simulink model "AirRefueling_Platform_ch10_WindGust"  (R2022a)
settings: Solver=ode3  StartTime=0.0  StopTime=270  FixedStep=0.01  RelTol=1e-5  AbsTol=1e-4  EnableMultiTasking=on
InitFcn:
  | F16_Init
values from neighbouring files (symbols this model uses):
  airSpeed = 393.72    [F16_Init.m]
  alpha0 = trimAlpha*180/pi    (= 6.62393794015)    [F16_Init.m]
  altitude = 9843    [F16_Init.m]
  b_ref = 30.0    (= 30)    [F16_Init.m]
  C = [ 1,0,0,zeros(1,15) ... (first row only)    [F16_Init.m]
  C2m = [C(1,:) ... (first row only)    [F16_Init.m]
  d_f_rc = [4.45;0;-3.81]    [F16_Init.m]
  d_pr_rc = [8.2;0.45;-3.3]    [F16_Init.m]
  dLEF = 0    [F16_Init.m]
  fi_flag = 1    [F16_Init.m]
  Kc = [ ... (first row only)    [F16_Init.m]
  Ki = zeros(4,3)    [F16_Init.m]
  Kp = zeros(4,18)    [F16_Init.m]
  mass = 636.94    [F16_Init.m]
  p0_pr = p0_rc + d_pr_rc    [F16_Init.m]
  p0_rc = [-28;0;0]    [F16_Init.m]
  trim_ail = 0.00874607850103852    (= 0.00874607850104)    [F16_Init.m]
  trim_control = [trim_thrust;trim_ele;trim_ail;trim_rud]    [F16_Init.m]
  trim_ele = -2.97973164860638    (= -2.97973164861)    [F16_Init.m]
  trim_rud = 0.0680302158182712    (= 0.0680302158183)    [F16_Init.m]
  trim_state1 = [trim_state;0;0;0;0;0;0]    [F16_Init.m]
  trim_thrust = 2279.08519954656    (= 2279.08519955)    [F16_Init.m]
  visual_err = [0;0;0]    [F16_Init.m]
undefined symbols (not defined in the file or in its folder): Cdr_, dockingPoint, dtheta10, dtheta20, F, height, k_reel, kd, l0, l1, l_density, Light, m0, Mdr, MIL, N, Rdr, Rl, STD, T_reel_initial, theta10, theta20, vt0
libraries: etargetslib x11, dspnetwork x10, aerolibconvert2 x6, aerolibasang x4, simulink x2, aerolibatmos2 x2, aerolibwind2 x2, aerolibobsolete x2, sharedtransform x2, aerolibutil x2, aerolibadyn x1, aerolibtransform2 x1
(part 1 of 3)
settings Model: Creator=WhisPer  LastModifiedBy=lzj
settings SolverCC: AutoScaleAbsTol=off  AlgebraicLoopSolver=TrustRegion
settings DataIOCC: LimitDataPoints=on  SaveFormat=Array  ReturnWorkspaceOutputs=off
settings OptimizationCC: LifeSpan=inf
settings DebuggingCC: UnderspecifiedInitializationDetection=Classic  MergeDetectMultiDrivingBlocksExec=none  SolverPrmCheckMsg=warning  InheritedTsInSrcMsg=none  ParameterPrecisionLossMsg=none  UnconnectedInputMsg=warning  UnconnectedOutputMsg=warning  UnconnectedLineMsg=warning  StateNameClashWarn=warning  SFUnexpectedBacktrackingDiag=warning  SFNoUnconditionalDefaultTransitionDiag=warning  SFExecutionAtInitializationDiag=none  SFMachineParentedDataDiag=warning  ArithmeticOperatorsInVariantConditions=warning
settings HardwareCC: ProdBitPerPointer=32  ProdBitPerSizeT=32  ProdBitPerPtrDiffT=32  ProdLargestAtomicFloat=None  ProdIntDivRoundTo=Undefined  ProdEndianess=Unspecified  ProdWordSize=32  ProdHWDeviceType=32-bit Generic
settings ModelReferenceCC: PropagateSignalLabelsOutOfModel=off
settings SFSimCC: SimUseLocalCustomCode=off  CustomCodeUndefinedFunction=UseInterfaceOnly
settings RTWCC: RTWUseLocalCustomCode=off  DLArmComputeVersion=19.05
settings CodeAppCC: StateflowObjectComments=on
settings GRTTargetCC: TargetLangStandard=C89/C90 (ANSI)
settings ConfigComp: CovMetricSettings=dw  CovSaveCumulativeToWorkspaceVar=on  CovSaveSingleToWorkspaceVar=on  CovExternalEMLEnable=off

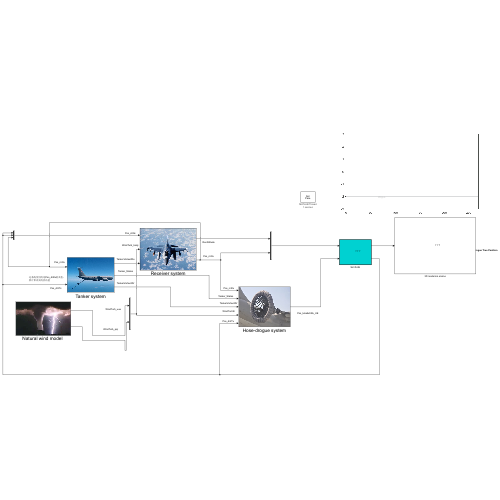
[thumbnail: Simulink's stored preview of the top-level diagram]
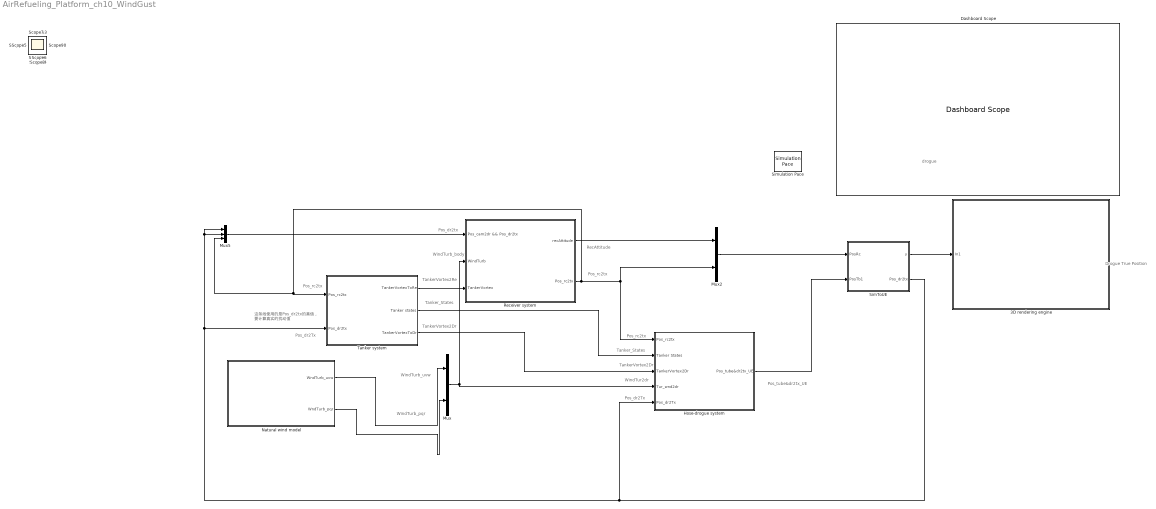
== system AirRefueling_Platform_ch10_WindGust ==
  note: 这条线使用的是Pos_dr2tx的真值，
      | 要计算真实的扰动值
  note: drogue
  note: RecAttitude
  note: WindTurb_uvw
  note: WindTurb_pqr
  note: Pos_tube&dr2tx_UE
  note: WindTur2dr
  note: WindTurb_body
  note: Pos_dr2tx
  note: Pos_rc2tx
  note: TankerVortex2Re
  note: TankerVortex2Dr
  note: Tanker_States
  note: Tanker_States
  note: TankerVortex2Dr
  note: Pos_rc2tx
  note: Drogue True Position
  note: Pos_dr2Tx
  note: Pos_rc2tx
  note: Pos_dr2Tx
  3D rendering engine : Subsystem
      mask Display: image('C:\Users\lgy13\Desktop\当下要完成的\AirRefueling3DVR-Blank\Icon\sideview.png'); % Use "Edit Image" on toolstrip to change.
  Dashboard Scope : DashboardScope
  Hose-drogue system : Subsystem
      mask Display: image(imread('Icon\drogue.jpg'))
  Mux : Mux  Inputs=2
  Mux2 : Mux  Inputs=2
  Mux5 : Mux  Inputs=3
  "Natural wind model " : Subsystem
      mask Display: image(imread('Icon\Enviroment.jpg'))
  Receiver system : Subsystem
      mask Display: image(imread('Icon\f16thumb.jpg'))
  SimToUE : MATLAB Function  TreatAsAtomicUnit=on
  Simulation Pace : aerolibanimutils/Simulation Pace  SimulationPace=1  SleepMode=MATLAB Thread  OutputPaceError=off  SampleTime=0.1
  Tanker system : Subsystem
      mask Display: image(imread('Icon\tanker.jpg'))
  Scope{,1,3..34} (34 alike) : Scope
  wires:
  SimToUE/2(Pos_dr2tx) -> Hose-drogue system/5(Pos_dr2Tx), Tanker system/2(Pos_dr2tx), Mux5/1, Mux5/2
  Receiver system/1(recAttitude) -> Mux2/1
  Hose-drogue system/1(Pos_tube&dr2tx_UE) -> SimToUE/2(PosTb1)
  Mux2/1 -> SimToUE/1(PosRc)
  Tanker system/2(Tanker states) -> Hose-drogue system/2(Tanker States)
  Tanker system/3(TankerVortexToDr) -> Hose-drogue system/3(TankerVortex2Dr)
  Tanker system/1(TankerVortexToRe) -> Receiver system/3(TankerVortex)
  Mux5/1 -> Receiver system/1(Pos_cam2dr && Pos_dr2tx)
  SimToUE/1(y) -> 3D rendering engine/1(In1)
  Receiver system/2(Pos_rc2tx) -> Mux2/2, Hose-drogue system/1(Pos_rc2tx), Mux5/3, Tanker system/1(Pos_rc2tx)
  "Natural wind model "/1(WndTurb_uvw) -> Mux/1
  "Natural wind model "/2(WndTurb_pqr) -> Mux/2
  Mux/1 -> Hose-drogue system/4(Tur_wnd2dr), Receiver system/2(WindTurb)

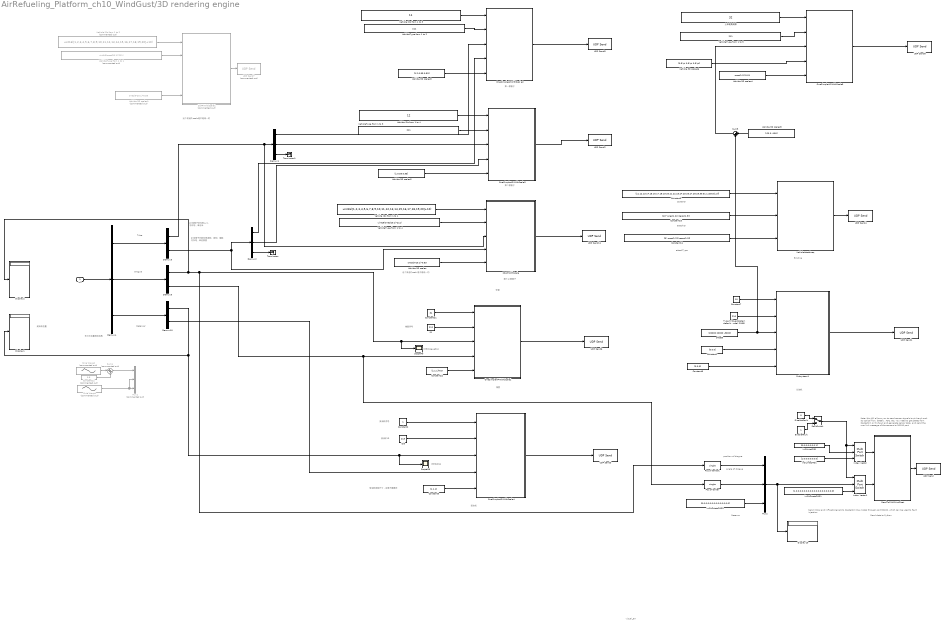
== system AirRefueling_Platform_ch10_WindGust/3D rendering engine ==
  note: visual_err
  note: 第一根管子
  note: 这个发送的scale是不是统一的
  note: 受油机位置
  note: 加油机
  note: 锥套
  note: position of drogue
  note: copterID
  note: Send inSILs and inFloats signals to CopterSim DLL model through port 30100, which can be used to fault injection.
  note: 记录RcPos
  note: 20段管子的位置xyz，
      | 北东地，单位米
  note: Note: this API allows you to send sensor signals to pixhawk such as optical flow, battery, ADC, etc. You need to get states from CopterSim or Pixhawk and generate sensor data, and send the mavlink message of the sensors to 30100 port
  note: 锥套序号
  note: attachType
  note: 记录DroguePos
  note: 受油机
  note: Tube
  note: 20段管子的欧拉角滚转、俯仰、偏航
      | 北东地，单位弧度
  note: attachID
  note: 先分为位置和欧拉角
  note: Binding
  note: Send data to Python
  note: Reserve
  note: 软管
  note: 受油机ID
  note: Drogue
  note: angle of drogue
  note: 受油机缩放尺寸，这里不需要改
  note: Receiver
  note: 受油机序号
  note: 这个发送的scale是不是统一的
  note: 第二根管子
  note: 剩下18根管子
  In1 : Inport
  20APIWithScale : Subsystem
  20APIWithScale1 : Subsystem  Commented=on
  Constant1 : Constant  Value=[0,0,0]
  Constant10 : Constant  Value=[10* ones(1,22),zeros(1,3)]
  Constant11 : Constant  Value=[3* ones(1,22),zeros(1,3)]
  Constant12 : Constant  Commented=on  Value=0.8
  Constant2 : Constant
  Constant21 : Constant  Value=31
  Constant22 : Constant  Value=[1,1,1]*0.5
  Constant3 : Constant  Value=[1,1,1]
  Constant7 : Constant  Value=10
  Constant8 : Constant  Value=[0,0,0]
  Constant9 : Constant  Value=[11,12,13,14,15,16,17,18,19,20,21,22,23,24,25,26,27,28,29,30,31,1,zeros(1,3)]
  Demux1 : Demux  Outputs=[3,3,54]
  Demux10 : Demux  Outputs=[3,3]
  Demux2 : Demux  Outputs=[3,3,54]
  Demux3 : Demux  Outputs=[60,60]
  Demux4 : Demux  Outputs=[120,6,6]
  Demux5 : Demux  Outputs=[3,3]
  DisableFault : Constant  Value=0
  Display1 : Display
  Display10 : Display
  Display2 : Display
  EnableFault : Constant
  FaultSwitch : ManualSwitch
  ID : Constant  Value=212
  ID3 : Constant  Value=213
  Index Vector : MultiPortSwitch  DataPortOrder=Zero-based contiguous  Inputs=2  zeroidx=on  SaturateOnIntegerOverflow=off  InputSameDT=off
  Index Vector1 : MultiPortSwitch  DataPortOrder=Zero-based contiguous  Inputs=2  zeroidx=on  SaturateOnIntegerOverflow=off  InputSameDT=off
  Mux1 : Mux  Commented=on  Inputs=3
  Mux2 : Mux  Inputs=[3 3 14]
  OneSimpleAPIWithScal e2 : Subsystem
  OneSimpleAPIWithScale1 : Subsystem
  OneSimpleAPIWithScale3 : Subsystem
  OneSimpleAPIWithScale4 : Subsystem
  OneSimpleAPIWithScale5 : Subsystem
  Pos of tanker : DataTypeConversion  OutDataTypeStr=single  SaturateOnIntegerOverflow=off  RndMeth=Floor
  Pos of tanker1 : DataTypeConversion  OutDataTypeStr=single  SaturateOnIntegerOverflow=off  RndMeth=Floor
  Scope38 : Scope
  Scope40 : Scope
  SendToPX4SILIntFloat : Subsystem
  Sine Wave1 : Sin  Commented=on  Amplitude=0  SampleTime=0
  Sine Wave2 : Sin  Commented=on  Amplitude=0.8  SampleTime=0
  Subsystem1 : Subsystem
  Sum4 : Sum  Commented=on  Inputs=|++
  Sum5 : Sum  Inputs=|++
  Terminator : Terminator
  Terminator1 : Terminator
  "Type 3 (Quadcopter), default model (F450)" : Constant  Value=210
  UDP Send : dspnetwork/UDP Send  remoteURL='224.0.0.10'  remotePort=20006  localURL='0.0.0.0'  localPortSource=Automatically determine  localPort=-1  sendBufferSize=8192  sampletime=-1  blockPlatform=[]  separateLengthPort=0
  UDP Send{1..6,8,11} (8 alike) : dspnetwork/UDP Send  remoteURL='127.0.0.1'  remotePort=20010  localURL='0.0.0.0'  localPortSource=Automatically determine  localPort=-1  sendBufferSize=8192  sampletime=-1  blockPlatform=[]  separateLengthPort=0
  UDP Send7 : dspnetwork/UDP Send  Commented=on  remoteURL='127.0.0.1'  remotePort=20010  localURL='0.0.0.0'  localPortSource=Automatically determine  localPort=-1  sendBufferSize=8192  sampletime=-1  blockPlatform=[]  separateLengthPort=0
  Vehicle 3D scales : Constant  Value=ones(3*20,1)*0.53
  Vehicle 3D scales1 : Constant  Commented=on  Value=ones(3*20,1)*0.53
  Vehicle 3D scales2 : Constant  Value=[1,0.53,0.53]
  Vehicle 3D scales3 : Constant  Value=[1.2,0.53,0.53]
  Vehicle 3D scales4 : Constant  Value=ones(1,3)*0.01
  Vehicle 3D scales5 : Constant  Value=[-20 0 -100]
  Vehicle 3D scales6 : Constant  Value=[0.5*pi 0.5*pi 0.5*pi]
  Vehicle IDs from 1 to 1 : Constant  Value=uint16([1,2,3,4,5,6,7,8,9,10,11,12,13,14,15,16,17,18,19,20]+10)
  Vehicle IDs from 1 to 2 : Constant  Commented=on  Value=uint16([1,2,3,4,5,6,7,8,9,10,11,12,13,14,15,16,17,18,19,20]+10)
  Vehicle IDs from 1 to 3 : Constant  Value=11
  Vehicle IDs from 1 to 4 : Constant  Value=12
  VehicleAttatchreq : Subsystem
  VehicleType from 1 to 1 : Constant  Commented=on  Value=uint16(ones(20,1)*211)
  VehicleType from 1 to 2 : Constant  Value=211
  VehicleType from 1 to 3 : Constant  Value=211
  VehicleType from 1 to 4 : Constant  Value=uint16(ones(20,1)*211)
  VehicleType from 1 to 5 : Constant  Value=211
  inSILFloatsCMD1 : Constant  Value=[1,0,0,0,0,0,0,0,0,0,0,0,0,0,0,0,0,0,0,0]  OutDataTypeStr=single
  inSILFloatsCMD3 : Constant  Value=[0,0,0,0,0,0,0,0,0,0,0,0,0,0]  OutDataTypeStr=single
  inSILIntsCMD : Constant  Value=[0,0,0,0,0,0,0,1]  OutDataTypeStr=int32
  inSILIntsCMD1 : Constant  Value=[1,0,0,0,0,0,0,0]  OutDataTypeStr=int32
  offset5 : Constant  Value=[20000 20000 -3000]
  上帝视角观察 : Constant  Value=32
  wires:
  inSILFloatsCMD3/1 -> Mux2/3
  Demux5/1 -> Display2/1, Pos of tanker1/1, Scope40/1, OneSimpleAPIWithScale1/3(PosE)
  Mux2/1 -> Display10/1, Index Vector1/2
  Constant11/1 -> VehicleAttatchreq/3(AttatchTypes)
  Constant1/1 -> Subsystem1/4(AngEuler)
  Constant10/1 -> VehicleAttatchreq/2(AttatchIDs)
  Constant9/1 -> VehicleAttatchreq/1(CopterIDs)
  DisableFault/1 -> FaultSwitch/1
  "Type 3 (Quadcopter), default model (F450)"/1 -> Subsystem1/2(vehicleType)  "VehicleType"
  In1/1 -> Demux4/1
  Constant21/1 -> OneSimpleAPIWithScale1/1(copterID)  "CopterID"
  OneSimpleAPIWithScale4/1(toUnReal) -> UDP Send3/1
  Pos of tanker1/1 -> Mux2/1
  Constant8/1 -> Subsystem1/5(VelE)
  20APIWithScale/1(Out1) -> UDP Send11/1
  Constant2/1 -> OneSimpleAPIWithScale4/1(copterID)  "CopterID"
  OneSimpleAPIWithScale1/1(toUnReal) -> UDP Send6/1
  Constant22/1 -> OneSimpleAPIWithScale1/5(ScaleXYZ)
  inSILIntsCMD/1 -> Index Vector/2
  Vehicle IDs from 1 to 1/1 -> 20APIWithScale/1(IDs)
  inSILIntsCMD1/1 -> Index Vector/3
  Constant3/1 -> OneSimpleAPIWithScale4/5(ScaleXYZ)
  Demux4/1 -> Demux3/1
  Constant7/1 -> Subsystem1/1(copterID)  "CopterID"
  FaultSwitch/1 -> Index Vector1/1, Index Vector/1
  Demux5/2 -> Pos of tanker/1, OneSimpleAPIWithScale1/4(AngEuler)
  Index Vector/1 -> SendToPX4SILIntFloat/1(inSILInts)
  ID/1 -> OneSimpleAPIWithScale1/2(vehicleType)  "VehicleType"
  Index Vector1/1 -> SendToPX4SILIntFloat/2(inSILFloats)
  Demux4/3 -> Demux10/1
  SendToPX4SILIntFloat/1(PX4SILIntFloat) -> UDP Send/1
  Demux10/2 -> OneSimpleAPIWithScale4/4(AngEuler)
  Subsystem1/1(toUnReal) -> UDP Send1/1
  ID3/1 -> OneSimpleAPIWithScale4/2(vehicleType)  "VehicleType"
  Pos of tanker/1 -> Mux2/2
  EnableFault/1 -> FaultSwitch/2
  inSILFloatsCMD1/1 -> Index Vector1/3
  VehicleType from 1 to 4/1 -> 20APIWithScale/2(VehileTypes)
  VehicleAttatchreq/1(Out1) -> UDP Send4/1
  Demux4/2 -> Demux5/1
  Demux3/1 -> Demux1/1, 20APIWithScale/3(PosEs)
  Sine Wave1/1 -> Mux1/2, Mux1/3
  Sum4/1 -> Mux1/1
  Constant12/1 -> Sum4/2
  Sine Wave2/1 -> Sum4/1
  Vehicle 3D scales/1 -> 20APIWithScale/5(scaleXYZ)
  OneSimpleAPIWithScale3/1(toUnReal) -> UDP Send2/1
  OneSimpleAPIWithScal e2/1(toUnReal) -> UDP Send5/1
  Vehicle IDs from 1 to 2/1 -> 20APIWithScale1/1(IDs)
  20APIWithScale1/1(Out1) -> UDP Send7/1
  VehicleType from 1 to 1/1 -> 20APIWithScale1/2(VehileTypes)
  Vehicle 3D scales1/1 -> 20APIWithScale1/5(scaleXYZ)
  Vehicle IDs from 1 to 3/1 -> OneSimpleAPIWithScal e2/1(copterID)
  VehicleType from 1 to 2/1 -> OneSimpleAPIWithScal e2/2(vehicleType)
  Vehicle IDs from 1 to 4/1 -> OneSimpleAPIWithScale3/1(copterID)
  VehicleType from 1 to 3/1 -> OneSimpleAPIWithScale3/2(vehicleType)
  Vehicle 3D scales3/1 -> OneSimpleAPIWithScal e2/5(ScaleXYZ)
  Vehicle 3D scales2/1 -> OneSimpleAPIWithScale3/5(ScaleXYZ)
  Demux1/1 -> OneSimpleAPIWithScal e2/3(PosE)
  Demux1/2 -> OneSimpleAPIWithScale3/3(PosE)
  Demux2/1 -> OneSimpleAPIWithScal e2/4(AngEuler)
  Demux2/2 -> OneSimpleAPIWithScale3/4(AngEuler)
  Demux3/2 -> Demux2/1, 20APIWithScale/4(AngEulers)
  Demux2/3 -> Terminator/1
  Demux1/3 -> Terminator1/1
  Demux10/1 -> Scope38/1, OneSimpleAPIWithScale4/3(PosE), Display1/1
  OneSimpleAPIWithScale5/1(toUnReal) -> UDP Send8/1
  上帝视角观察/1 -> OneSimpleAPIWithScale5/1(copterID)
  Vehicle 3D scales4/1 -> OneSimpleAPIWithScale5/5(ScaleXYZ)
  VehicleType from 1 to 5/1 -> OneSimpleAPIWithScale5/2(vehicleType)
  Vehicle 3D scales6/1 -> OneSimpleAPIWithScale5/4(AngEuler)
  offset5/1 -> Sum5/2, Subsystem1/3(PosE)
  Vehicle 3D scales5/1 -> Sum5/1
  Sum5/1 -> OneSimpleAPIWithScale5/3(PosE)

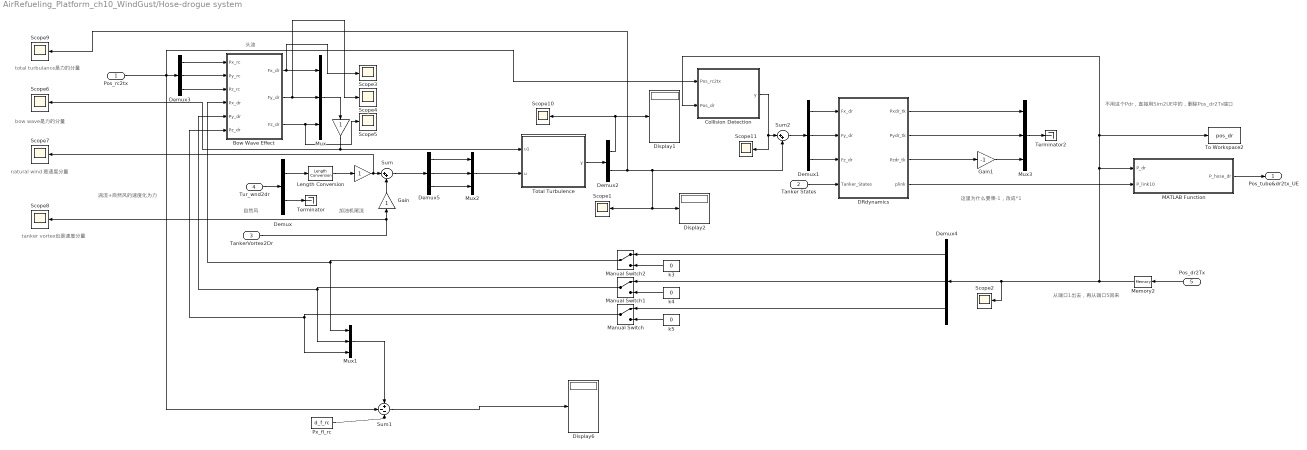
== system AirRefueling_Platform_ch10_WindGust/Hose-drogue system ==
  note: 从端口1出去，再从端口5回来
  note: 不用这个Pdr，直接用Sim2UE中的，删除Pos_dr2Tx端口
  note: 涡流+自然风的速度化为力
  note: total turbulance是力的分量
  note: tanker vortex也是速度分量
  note: natural wind 是速度分量
  note: bow wave是力的分量
  note: 自然风
  note: 加油机尾流
  note: 头波
  note: 这里为什么要乘-1，改成*1
  Pos_rc2tx : Inport
  Tanker States : Inport  Port=2
  TankerVortex2Dr : Inport  Port=3
  Tur_wnd2dr : Inport  Port=4
  Pos_dr2Tx : Inport  Port=5
  " " : Gain
  "  " : Gain
  Bow Wave Effect : Subsystem
  Collision Detection : Subsystem
  DRdynamics : Subsystem
  Demux : Demux  Outputs=2
  Demux1 : Demux  Outputs=3
  Demux2 : Demux  Outputs=[3,3]
  Demux3 : Demux  Outputs=3
  Demux4 : Demux  Outputs=3
  Demux5 : Demux  Outputs=[1,1,1]
  Display1 : Display
  Display2 : Display
  Display6 : Display
  Gain : Gain
  Gain1 : Gain  Gain=-1
  Length Conversion : aerolibconvert2/Length Conversion  IU=ft  OU=m
  MATLAB Function : MATLAB Function  TreatAsAtomicUnit=on
  Manual Switch : ManualSwitch
  Manual Switch1 : ManualSwitch
  Manual Switch2 : ManualSwitch
  Memory2 : Memory  InitialCondition=l1
  Mux : Mux  Inputs=3
  Mux1 : Mux  Inputs=3
  Mux2 : Mux  Inputs=[1,1,1]
  Mux3 : Mux  Inputs=3
  Px_fl_rc : Constant  Value=d_f_rc
  Scope{1..11} (11 alike) : Scope
  Sum : Sum  Inputs=|++
  Sum1 : Sum  Inputs=+--
  Sum2 : Sum  Inputs=|++
  Terminator : Terminator
  Terminator2 : Terminator
  To Workspace2 : ToWorkspace  VariableName=pos_dr  SampleTime=-1
  "Total Turbulence  " : MATLAB Function  TreatAsAtomicUnit=on
  k3 : Constant  Value=0
  k4 : Constant  Value=0
  k5 : Constant  Value=0
  Pos_tube&dr2tx_UE : Outport
  wires:
  Mux/1 -> "  "/1
  TankerVortex2Dr/1 -> Scope8/1, Gain/1
  Demux/1 -> Length Conversion/1
  Demux1/3 -> DRdynamics/3(Fz_dr)
  Demux1/2 -> DRdynamics/2(Fy_dr)
  Demux1/1 -> DRdynamics/1(Fx_dr)
  Demux/2 -> Terminator/1
  Tur_wnd2dr/1 -> Demux/1
  Bow Wave Effect/3(Fz_dr) -> Scope5/1, Mux/3
  Bow Wave Effect/2(Fy_dr) -> Scope4/1, Mux/2
  Bow Wave Effect/1(Fx_dr) -> Scope3/1, Mux/1
  Demux3/1 -> Bow Wave Effect/1(Px_rc)
  k4/1 -> Manual Switch1/2
  Manual Switch1/1 -> Mux1/2, Bow Wave Effect/5(Py_dr)
  Manual Switch2/1 -> Mux1/1, Bow Wave Effect/4(Px_dr)
  k5/1 -> Manual Switch/2
  k3/1 -> Manual Switch2/2
  Manual Switch/1 -> Mux1/3, Bow Wave Effect/6(Pz_dr)
  DRdynamics/2(Pydr_tk) -> Mux3/2
  DRdynamics/1(Pxdr_tk) -> Mux3/1
  Gain1/1 -> Mux3/3
  DRdynamics/3(Pzdr_tk) -> Gain1/1
  Demux3/3 -> Bow Wave Effect/3(Pz_rc)
  Demux3/2 -> Bow Wave Effect/2(Py_rc)
  "Total Turbulence  "/1(y) -> Demux2/1
  DRdynamics/4(plink) -> MATLAB Function/2(P_link10)
  Gain/1 -> Sum/2
  " "/1 -> Scope7/1, Sum/1
  "  "/1 -> "Total Turbulence  "/1(u1), Scope6/1
  Tanker States/1 -> DRdynamics/4(Tanker_States)
  Length Conversion/1 -> " "/1
  Mux1/1 -> Sum1/1
  Px_fl_rc/1 -> Sum1/3
  Pos_rc2tx/1 -> Collision Detection/1(Pos_rc2tx), Sum1/2, Demux3/1
  Sum1/1 -> Display6/1
  Demux2/2 -> Scope9/1, Sum2/2, Scope1/1, Display2/1
  Demux2/1 -> Display1/1, Scope10/1
  Collision Detection/1(y) -> Sum2/1, Scope11/1
  Sum2/1 -> Demux1/1
  MATLAB Function/1(P_hose_dr) -> Pos_tube&dr2tx_UE/1
  Pos_dr2Tx/1 -> Memory2/1
  Demux4/1 -> Manual Switch2/1
  Demux4/2 -> Manual Switch1/1
  Demux4/3 -> Manual Switch/1
  Mux3/1 -> Terminator2/1
  Memory2/1 -> Scope2/1, Demux4/1, Collision Detection/2(Pos_dr), To Workspace2/1, MATLAB Function/1(P_dr)
  Sum/1 -> Demux5/1
  Demux5/2 -> Mux2/2
  Demux5/3 -> Mux2/3
  Demux5/1 -> Mux2/1
  Mux2/1 -> "Total Turbulence  "/2(u)

== system AirRefueling_Platform_ch10_WindGust/Natural wind model  ==
  Discrete Wind Gust Model - On : aerolibwind2/Discrete Wind Gust Model  units=Metric (MKS)  Gx=on  Gy=on  Gz=on  t_0=100  d_m=[120 120 80]  v_m=[0 5 5]
  Display1 : Display
  Display2 : Display
  Dot Product2 : DotProduct  SaturateOnIntegerOverflow=on  InputSameDT=off  OutDataTypeStr=Inherit: Inherit via internal rule
  Dryden Wind Turbulence Model (Continuous (+q -r)) : aerolibwind2/Dryden Wind Turbulence Model  (Continuous (+q -r))  units=Metric (MKS)  spec=MIL-F-8785C  model=Continuous Dryden (+q -r)  W20=5  Wdeg=0  TurbProb=10^-2 - Light  L_high=533.5  Wingspan=6  ts=0.01  Seed=1+fix(36500*rand(1,4))  T_on=on
  Model Info : simulink/Model-Wide Utilities/Model Info  Frame=on  DisplayStringWithTags=|  HorizontalTextAlignment=Center  LeftAlignmentValue=0.5
      | The resultant mean wind speed and angular rates is in the body-fixed axis. 
      | The simulation parameter is set to
      | altitude:3000m
      | airspeed:120m/s
  Scope1 : Scope
  Scope2 : Scope
  Scope3 : Scope
  Sum : Sum  Inputs=|++  InputSameDT=on  SaturateOnIntegerOverflow=on  OutDataTypeStr=Inherit: Same as first input
  V2 : Math  Operator=sqrt  SignedPower=on
  constan1 : Constant  Value=airSpeed
  constant : Constant  Value=altitude
  WndTurb_uvw : Outport
  WndTurb_pqr : Outport  Port=2
  wires:
  [DCM] -> Dryden Wind Turbulence Model (Continuous (+q -r))/3
  V2/1 -> Dryden Wind Turbulence Model (Continuous (+q -r))/2, Discrete Wind Gust Model - On/1
  Dot Product2/1 -> V2/1
  constan1/1 -> Dot Product2/1, Dot Product2/2, Display1/1
  Discrete Wind Gust Model - On/1 -> Sum/2
  Dryden Wind Turbulence Model (Continuous (+q -r))/2 -> Scope1/1, WndTurb_pqr/1
  Dryden Wind Turbulence Model (Continuous (+q -r))/1 -> Scope3/1, Sum/1
  constant/1 -> Display2/1, Dryden Wind Turbulence Model (Continuous (+q -r))/1
  Sum/1 -> Scope2/1, WndTurb_uvw/1

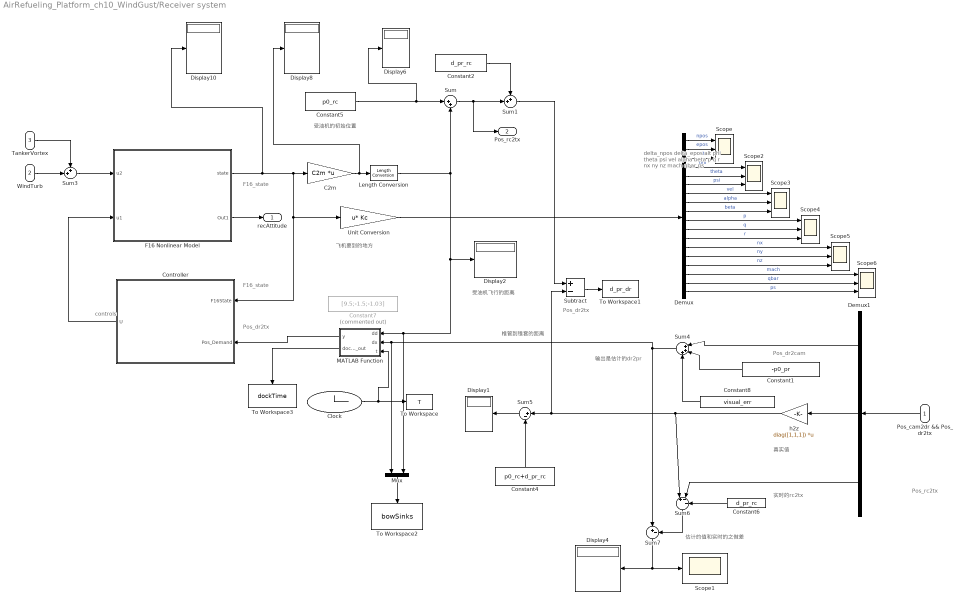
== system AirRefueling_Platform_ch10_WindGust/Receiver system ==
  note: 估计的值和实时的之做差
  note: 实时的rc2tx
  note: Pos_rc2tx
  note: 输出是估计的dr2pr
  note: 真实值
  note: Pos_dr2cam
  note: 飞机要到的地方
  note: 受油机的初始位置
  note: 受油机飞行的距离
  note: 椎管到锥套的距离
  note: controls
  note: Pos_dr2tx
  note: F16_state
  note: delta_npos
      | delta_epos
      | alt
      | phi
      | theta
      | psi
      | vel
      | alpha
      | beta
      | p
      | q
      | r
      | nx
      | ny
      | nz
      | mach
      | qbar
      | ps
  note: F16_state
  note: Pos_dr2tx
  Pos_cam2dr && Pos_dr2tx : Inport
  WindTurb : Inport  Port=2
  TankerVortex : Inport  Port=3
  C2m : Gain  Gain=C2m  Multiplication=Matrix(K*u) (u vector)
  Clock : Clock
      settings: Decimation=50
  Constant1 : Constant  Value=-p0_pr
  Constant2 : Constant  Value=d_pr_rc
  Constant4 : Constant  Value=p0_rc+d_pr_rc
  Constant5 : Constant  Value=p0_rc
  Constant6 : Constant  Value=d_pr_rc
  Constant7 : Constant  Commented=on  Value=[9.5;-1.5;-1.03]
  Constant8 : Constant  Value=visual_err
  Controller : Subsystem
      mask Display: image(imread('Icon\F16_Pilot.jpg'))
  Demux : Demux  Outputs=18
      settings: DisplayOption=none
  Demux1 : Demux  Outputs=[3,3,3]
  Display{1..2,4,6,8,10} (6 alike) : Display
  F16 Nonlinear Model : Subsystem
      mask Display: image(imread('Icon\fighter_f16.jpg'))
  Length Conversion : aerolibconvert2/Length Conversion  IU=ft  OU=m
  MATLAB Function : MATLAB Function  TreatAsAtomicUnit=on
  Mux : Mux  Inputs=2
  Scope{,2..6} (6 alike) : Scope  NumInputPorts=3
  Scope1 : Scope
  Subtract : Sum  Inputs=+-
  Sum : Sum  Inputs=|++
  Sum1 : Sum  Inputs=++|
  Sum3 : Sum  Inputs=++|
  Sum4 : Sum  Inputs=|+++
  Sum5 : Sum  Inputs=|+-
  Sum6 : Sum  Inputs=|+--
  Sum7 : Sum  Inputs=|+-
  To Workspace : ToWorkspace  VariableName=T  SampleTime=-1
      settings: Decimation=100
  To Workspace1 : ToWorkspace  VariableName=d_pr_dr  SampleTime=-1
  To Workspace2 : ToWorkspace  VariableName=bowSinks  SampleTime=-1
  To Workspace3 : ToWorkspace  VariableName=dockTime  SampleTime=-1
      settings: Save2DSignal=2-D array (concatenate along first dimension)
  Unit Conversion : Gain  Gain=Kc  Multiplication=Matrix(u*K)
  h2z : Gain  Gain=diag([1,1,1])  Multiplication=Matrix(K*u)
  recAttitude : Outport
  Pos_rc2tx : Outport  Port=2
  wires:
  Clock/1 -> MATLAB Function/3(t), To Workspace/1
  WindTurb/1 -> Sum3/2
  F16 Nonlinear Model/1(state) -> Display10/1, C2m/1, Controller/1(F16State), Unit Conversion/1
  Demux/1 -> Scope/1  "npos"
  Demux/2 -> Scope/2  "epos"
  Demux/3 -> Scope/3  "alt"
  Demux/5 -> Scope2/2  "theta"
  Demux/6 -> Scope2/3  "psi"
  Demux/7 -> Scope3/1  "vel"
  Demux/8 -> Scope3/2  "alpha"
  Demux/9 -> Scope3/3  "beta"
  Demux/10 -> Scope4/1  "p"
  Demux/11 -> Scope4/2  "q"
  Demux/12 -> Scope4/3  "r"
  Demux/13 -> Scope5/1  "nx"
  Demux/14 -> Scope5/2  "ny"
  Demux/15 -> Scope5/3  "nz"
  Demux/4 -> Scope2/1  "phi"
  Demux/16 -> Scope6/1  "mach"
  Demux/17 -> Scope6/2  "qbar"
  Demux/18 -> Scope6/3  "ps"
  Unit Conversion/1 -> Demux/1
  F16 Nonlinear Model/2(Out1) -> recAttitude/1
  C2m/1 -> Display8/1, Length Conversion/1
  Sum3/1 -> F16 Nonlinear Model/1(u2)
  TankerVortex/1 -> Sum3/1
  Length Conversion/1 -> MATLAB Function/1(dd), Mux/2, Display2/1, Sum/2
  Constant1/1 -> Sum4/2
  Pos_cam2dr && Pos_dr2tx/1 -> Demux1/1
  Constant2/1 -> Sum1/1
  Subtract/1 -> To Workspace1/1
  Controller/1(U) -> F16 Nonlinear Model/2(u1)
  Sum/1 -> Pos_rc2tx/1, Sum1/2
  Demux1/2 -> h2z/1
  h2z/1 -> Sum6/1, Sum5/1, Subtract/2
  Sum4/1 -> Sum7/1, Mux/1, MATLAB Function/2(dx)
  Sum5/1 -> Display1/1
  Constant4/1 -> Sum5/2
  Sum7/1 -> Scope1/1, Display4/1
  Constant6/1 -> Sum6/3
  Sum6/1 -> Sum7/2
  Demux1/1 -> Sum4/1
  Demux1/3 -> Sum6/2
  Sum1/1 -> Subtract/1
  MATLAB Function/1(y) -> Controller/2(Pos_Demand)
  Constant8/1 -> Sum4/3
  Constant5/1 -> Display6/1, Sum/1
  Mux/1 -> To Workspace2/1
  MATLAB Function/2(dockTime_out) -> To Workspace3/1

== system AirRefueling_Platform_ch10_WindGust/Tanker system ==
  note: pt
  note: vt
  note: al
  Pos_rc2tx : Inport
  Pos_dr2tx : Inport  Port=2
  " " : MATLAB Function  TreatAsAtomicUnit=on
  "  " : MATLAB Function  TreatAsAtomicUnit=on
  Demux : Demux  Outputs=2
  Display1 : Display
  Display3 : Display
  Integrator : Integrator  InitialCondition=vt0
  Integrator1 : Integrator  InitialCondition=[0;0;0]
  Length Conversion : aerolibconvert2/Length Conversion  IU=m  OU=ft
  Mux : Mux  Inputs=3
  Mux1 : Mux  Inputs=2
  tanker acceleration : Constant  Value=[0;0;0]
  TankerVortexToRe : Outport
  Tanker states : Outport  Port=2
  TankerVortexToDr : Outport  Port=3
  wires:
  tanker acceleration/1 -> Mux/3, Integrator/1
  Integrator/1 -> Mux/2, Integrator1/1
  Mux/1 -> Tanker states/1
  Pos_dr2tx/1 -> Display1/1, "  "/1(u)
  "  "/1(y) -> TankerVortexToDr/1
  Integrator1/1 -> Mux/1
  " "/1(y) -> Demux/1
  Mux1/1 -> TankerVortexToRe/1
  Demux/2 -> Mux1/2
  Length Conversion/1 -> Mux1/1
  Demux/1 -> Length Conversion/1
  Pos_rc2tx/1 -> Display3/1, " "/1(u)

== system AirRefueling_Platform_ch10_WindGust/3D rendering engine/20APIWithScale ==
  note: struct Multi3DData1New {
      |        int checksum;
      | 	uint16 IDs[20];
      | 	uint16 VehileTypes[20];
      | 	float PosE[60];
      | 	float AngEuler[60];
      | 	uint16 ScaleXYZ[60];
      | }
  note: scale value * 100
  IDs : Inport  PortDimensions=20
  VehileTypes : Inport  Port=2  PortDimensions=20
  PosEs : Inport  Port=3  PortDimensions=60
  AngEulers : Inport  Port=4  PortDimensions=60
  scaleXYZ : Inport  Port=5  PortDimensions=60
  Constant7 : Constant  Value=1234567890
  Data Type Conversion : DataTypeConversion  OutDataTypeStr=uint16  SaturateOnIntegerOverflow=off  RndMeth=Floor
  Data Type Conversion1 : DataTypeConversion  OutDataTypeStr=uint16  SaturateOnIntegerOverflow=off  RndMeth=Floor
  Data Type Conversion2 : DataTypeConversion  OutDataTypeStr=single  SaturateOnIntegerOverflow=off  RndMeth=Floor
  Data Type Conversion3 : DataTypeConversion  OutDataTypeStr=single  SaturateOnIntegerOverflow=off  RndMeth=Floor
  Data Type Conversion4 : DataTypeConversion  OutDataTypeStr=uint16  SaturateOnIntegerOverflow=off  RndMeth=Floor
  Data Type Conversion5 : DataTypeConversion  OutDataTypeStr=int32  SaturateOnIntegerOverflow=off  RndMeth=Floor
  Gain : Gain  Gain=100
  PayLoad : etargetslib/Byte Pack  datatypes={'int32','uint16','uint16','single','single','uint16'}  byteAlign=4
  Saturation : Saturate  UpperLimit=655.35  LowerLimit=0.01
  Out1 : Outport  VectorParamsAs1DForOutWhenUnconnected=off
  wires:
  Data Type Conversion3/1 -> PayLoad/5
  Data Type Conversion1/1 -> PayLoad/3
  PosEs/1 -> Data Type Conversion2/1
  Data Type Conversion2/1 -> PayLoad/4
  AngEulers/1 -> Data Type Conversion3/1
  PayLoad/1 -> Out1/1
  VehileTypes/1 -> Data Type Conversion1/1
  Data Type Conversion/1 -> PayLoad/2
  IDs/1 -> Data Type Conversion/1
  scaleXYZ/1 -> Saturation/1
  Data Type Conversion4/1 -> PayLoad/6
  Saturation/1 -> Gain/1
  Gain/1 -> Data Type Conversion4/1
  Constant7/1 -> Data Type Conversion5/1
  Data Type Conversion5/1 -> PayLoad/1

== system AirRefueling_Platform_ch10_WindGust/3D rendering engine/20APIWithScale1 ==
  note: struct Multi3DData1New {
      |        int checksum;
      | 	uint16 IDs[20];
      | 	uint16 VehileTypes[20];
      | 	float PosE[60];
      | 	float AngEuler[60];
      | 	uint16 ScaleXYZ[60];
      | }
  note: scale value * 100
  IDs : Inport  PortDimensions=20
  VehileTypes : Inport  Port=2  PortDimensions=20
  PosEs : Inport  Port=3  PortDimensions=60
  AngEulers : Inport  Port=4  PortDimensions=60
  scaleXYZ : Inport  Port=5  PortDimensions=60
  Constant7 : Constant  Value=1234567890
  Data Type Conversion : DataTypeConversion  OutDataTypeStr=uint16  SaturateOnIntegerOverflow=off  RndMeth=Floor
  Data Type Conversion1 : DataTypeConversion  OutDataTypeStr=uint16  SaturateOnIntegerOverflow=off  RndMeth=Floor
  Data Type Conversion2 : DataTypeConversion  OutDataTypeStr=single  SaturateOnIntegerOverflow=off  RndMeth=Floor
  Data Type Conversion3 : DataTypeConversion  OutDataTypeStr=single  SaturateOnIntegerOverflow=off  RndMeth=Floor
  Data Type Conversion4 : DataTypeConversion  OutDataTypeStr=uint16  SaturateOnIntegerOverflow=off  RndMeth=Floor
  Data Type Conversion5 : DataTypeConversion  OutDataTypeStr=int32  SaturateOnIntegerOverflow=off  RndMeth=Floor
  Gain : Gain  Gain=100
  PayLoad : etargetslib/Byte Pack  datatypes={'int32','uint16','uint16','single','single','uint16'}  byteAlign=4
  Saturation : Saturate  UpperLimit=655.35  LowerLimit=0.01
  Out1 : Outport  VectorParamsAs1DForOutWhenUnconnected=off
  wires:
  Data Type Conversion3/1 -> PayLoad/5
  Data Type Conversion1/1 -> PayLoad/3
  PosEs/1 -> Data Type Conversion2/1
  Data Type Conversion2/1 -> PayLoad/4
  AngEulers/1 -> Data Type Conversion3/1
  PayLoad/1 -> Out1/1
  VehileTypes/1 -> Data Type Conversion1/1
  Data Type Conversion/1 -> PayLoad/2
  IDs/1 -> Data Type Conversion/1
  scaleXYZ/1 -> Saturation/1
  Data Type Conversion4/1 -> PayLoad/6
  Saturation/1 -> Gain/1
  Gain/1 -> Data Type Conversion4/1
  Constant7/1 -> Data Type Conversion5/1
  Data Type Conversion5/1 -> PayLoad/1

== system AirRefueling_Platform_ch10_WindGust/3D rendering engine/OneSimpleAPIWithScal e2 ==
  note: //输出到模拟器的数据
      | struct SOut2SimulatorSimple1 {
      | 	int checkSum;
      | 	int copterID;  //Vehicle ID
      | 	int vehicleType;  //Vehicle type
      | 	float MotorRPMSMean;
      | 	float PosE[3];   //NED vehicle position in earth frame (m)
      | 	float AngEuler[3];  //Vehicle Euler angle roll pitch yaw (rad) in x y z
      | 	float Scale[3];
      | }
  note: All acutators will use this value
  copterID : Inport  PortDimensions=1
  vehicleType : Inport  Port=2  PortDimensions=1
  PosE : Inport  Port=3  PortDimensions=3
  AngEuler : Inport  Port=4  PortDimensions=3
  ScaleXYZ : Inport  Port=5  PortDimensions=3
  Constant7 : Constant  Value=1234567890
  Data Type Conversion : DataTypeConversion  OutDataTypeStr=int32  SaturateOnIntegerOverflow=off  RndMeth=Floor
  Data Type Conversion1 : DataTypeConversion  OutDataTypeStr=single  SaturateOnIntegerOverflow=off  RndMeth=Floor
  Mux : Mux  Inputs=3
  Mux1 : Mux
  PWMs : Constant  Value=3000
  PayLoad : etargetslib/Byte Pack  datatypes={'int32','single'}  byteAlign=1
  toUnReal : Outport  VectorParamsAs1DForOutWhenUnconnected=off
  wires:
  PayLoad/1 -> toUnReal/1
  Data Type Conversion/1 -> PayLoad/1
  Data Type Conversion1/1 -> PayLoad/2
  copterID/1 -> Mux/2
  vehicleType/1 -> Mux/3
  Constant7/1 -> Mux/1
  Mux/1 -> Data Type Conversion/1
  Mux1/1 -> Data Type Conversion1/1
  PWMs/1 -> Mux1/1
  PosE/1 -> Mux1/2
  AngEuler/1 -> Mux1/3
  ScaleXYZ/1 -> Mux1/4

== system AirRefueling_Platform_ch10_WindGust/3D rendering engine/OneSimpleAPIWithScale1 ==
  note: //输出到模拟器的数据
      | struct SOut2SimulatorSimple1 {
      | 	int checkSum;
      | 	int copterID;  //Vehicle ID
      | 	int vehicleType;  //Vehicle type
      | 	float MotorRPMSMean;
      | 	float PosE[3];   //NED vehicle position in earth frame (m)
      | 	float AngEuler[3];  //Vehicle Euler angle roll pitch yaw (rad) in x y z
      | 	float Scale[3];
      | }
  note: All acutators will use this value
  copterID : Inport  PortDimensions=1
  vehicleType : Inport  Port=2  PortDimensions=1
  PosE : Inport  Port=3  PortDimensions=3
  AngEuler : Inport  Port=4  PortDimensions=3
  ScaleXYZ : Inport  Port=5  PortDimensions=3
  Constant7 : Constant  Value=1234567890
  Data Type Conversion : DataTypeConversion  OutDataTypeStr=int32  SaturateOnIntegerOverflow=off  RndMeth=Floor
  Data Type Conversion1 : DataTypeConversion  OutDataTypeStr=single  SaturateOnIntegerOverflow=off  RndMeth=Floor
  Mux : Mux  Inputs=3
  Mux1 : Mux
  PWMs : Constant  Value=3000
  PayLoad : etargetslib/Byte Pack  datatypes={'int32','single'}  byteAlign=1
  toUnReal : Outport  VectorParamsAs1DForOutWhenUnconnected=off
  wires:
  PayLoad/1 -> toUnReal/1
  Data Type Conversion/1 -> PayLoad/1
  Data Type Conversion1/1 -> PayLoad/2
  copterID/1 -> Mux/2
  vehicleType/1 -> Mux/3
  Constant7/1 -> Mux/1
  Mux/1 -> Data Type Conversion/1
  Mux1/1 -> Data Type Conversion1/1
  PWMs/1 -> Mux1/1
  PosE/1 -> Mux1/2
  AngEuler/1 -> Mux1/3
  ScaleXYZ/1 -> Mux1/4

== system AirRefueling_Platform_ch10_WindGust/3D rendering engine/OneSimpleAPIWithScale3 ==
  note: All acutators will use this value
  note: //输出到模拟器的数据
      | struct SOut2SimulatorSimple1 {
      | 	int checkSum;
      | 	int copterID;  //Vehicle ID
      | 	int vehicleType;  //Vehicle type
      | 	float MotorRPMSMean;
      | 	float PosE[3];   //NED vehicle position in earth frame (m)
      | 	float AngEuler[3];  //Vehicle Euler angle roll pitch yaw (rad) in x y z
      | 	float Scale[3];
      | }
  copterID : Inport  PortDimensions=1
  vehicleType : Inport  Port=2  PortDimensions=1
  PosE : Inport  Port=3  PortDimensions=3
  AngEuler : Inport  Port=4  PortDimensions=3
  ScaleXYZ : Inport  Port=5  PortDimensions=3
  Constant7 : Constant  Value=1234567890
  Data Type Conversion : DataTypeConversion  OutDataTypeStr=int32  SaturateOnIntegerOverflow=off  RndMeth=Floor
  Data Type Conversion1 : DataTypeConversion  OutDataTypeStr=single  SaturateOnIntegerOverflow=off  RndMeth=Floor
  Mux : Mux  Inputs=3
  Mux1 : Mux
  PWMs : Constant  Value=3000
  PayLoad : etargetslib/Byte Pack  datatypes={'int32','single'}  byteAlign=1
  toUnReal : Outport  VectorParamsAs1DForOutWhenUnconnected=off
  wires:
  ScaleXYZ/1 -> Mux1/4
  AngEuler/1 -> Mux1/3
  PosE/1 -> Mux1/2
  PWMs/1 -> Mux1/1
  Mux1/1 -> Data Type Conversion1/1
  Mux/1 -> Data Type Conversion/1
  Constant7/1 -> Mux/1
  vehicleType/1 -> Mux/3
  copterID/1 -> Mux/2
  Data Type Conversion1/1 -> PayLoad/2
  Data Type Conversion/1 -> PayLoad/1
  PayLoad/1 -> toUnReal/1

== system AirRefueling_Platform_ch10_WindGust/3D rendering engine/OneSimpleAPIWithScale4 ==
  note: All acutators will use this value
  note: //输出到模拟器的数据
      | struct SOut2SimulatorSimple1 {
      | 	int checkSum;
      | 	int copterID;  //Vehicle ID
      | 	int vehicleType;  //Vehicle type
      | 	float MotorRPMSMean;
      | 	float PosE[3];   //NED vehicle position in earth frame (m)
      | 	float AngEuler[3];  //Vehicle Euler angle roll pitch yaw (rad) in x y z
      | 	float Scale[3];
      | }
  copterID : Inport  PortDimensions=1
  vehicleType : Inport  Port=2  PortDimensions=1
  PosE : Inport  Port=3  PortDimensions=3
  AngEuler : Inport  Port=4  PortDimensions=3
  ScaleXYZ : Inport  Port=5  PortDimensions=3
  Constant7 : Constant  Value=1234567890
  Data Type Conversion : DataTypeConversion  OutDataTypeStr=int32  SaturateOnIntegerOverflow=off  RndMeth=Floor
  Data Type Conversion1 : DataTypeConversion  OutDataTypeStr=single  SaturateOnIntegerOverflow=off  RndMeth=Floor
  Mux : Mux  Inputs=3
  Mux1 : Mux
  PWMs : Constant  Value=3000
  PayLoad : etargetslib/Byte Pack  datatypes={'int32','single'}  byteAlign=1
  toUnReal : Outport  VectorParamsAs1DForOutWhenUnconnected=off
  wires:
  ScaleXYZ/1 -> Mux1/4
  AngEuler/1 -> Mux1/3
  PosE/1 -> Mux1/2
  PWMs/1 -> Mux1/1
  Mux1/1 -> Data Type Conversion1/1
  Mux/1 -> Data Type Conversion/1
  Constant7/1 -> Mux/1
  vehicleType/1 -> Mux/3
  copterID/1 -> Mux/2
  Data Type Conversion1/1 -> PayLoad/2
  Data Type Conversion/1 -> PayLoad/1
  PayLoad/1 -> toUnReal/1

== system AirRefueling_Platform_ch10_WindGust/3D rendering engine/OneSimpleAPIWithScale5 ==
  note: //输出到模拟器的数据
      | struct SOut2SimulatorSimple1 {
      | 	int checkSum;
      | 	int copterID;  //Vehicle ID
      | 	int vehicleType;  //Vehicle type
      | 	float MotorRPMSMean;
      | 	float PosE[3];   //NED vehicle position in earth frame (m)
      | 	float AngEuler[3];  //Vehicle Euler angle roll pitch yaw (rad) in x y z
      | 	float Scale[3];
      | }
  note: All acutators will use this value
  copterID : Inport  PortDimensions=1
  vehicleType : Inport  Port=2  PortDimensions=1
  PosE : Inport  Port=3  PortDimensions=3
  AngEuler : Inport  Port=4  PortDimensions=3
  ScaleXYZ : Inport  Port=5  PortDimensions=3
  Constant7 : Constant  Value=1234567890
  Data Type Conversion : DataTypeConversion  OutDataTypeStr=int32  SaturateOnIntegerOverflow=off  RndMeth=Floor
  Data Type Conversion1 : DataTypeConversion  OutDataTypeStr=single  SaturateOnIntegerOverflow=off  RndMeth=Floor
  Mux : Mux  Inputs=3
  Mux1 : Mux
  PWMs : Constant  Value=3000
  PayLoad : etargetslib/Byte Pack  datatypes={'int32','single'}  byteAlign=1
  toUnReal : Outport  VectorParamsAs1DForOutWhenUnconnected=off
  wires:
  PayLoad/1 -> toUnReal/1
  Data Type Conversion/1 -> PayLoad/1
  Data Type Conversion1/1 -> PayLoad/2
  copterID/1 -> Mux/2
  vehicleType/1 -> Mux/3
  Constant7/1 -> Mux/1
  Mux/1 -> Data Type Conversion/1
  Mux1/1 -> Data Type Conversion1/1
  PWMs/1 -> Mux1/1
  PosE/1 -> Mux1/2
  AngEuler/1 -> Mux1/3
  ScaleXYZ/1 -> Mux1/4

== system AirRefueling_Platform_ch10_WindGust/3D rendering engine/SendToPX4SILIntFloat ==
  note: struct PX4SILIntFloat {
      | int checksum ;
      | int CopterID ;
      | int inSILInts [ 8 ];
      | float inSILFLoats [ 20 ];
      | }
  note: This message will be sent to PX4 DLL model's input signals inSILInts[8] and inSILFloats[20].
      | The checksum should be set to 1234567897, and the data should be sent to port 30100+(i-1)*2
  inSILInts : Inport  OutDataTypeStr=int32  PortDimensions=8
  inSILFloats : Inport  Port=2  OutDataTypeStr=single  PortDimensions=20
  CopterID : Constant  Value=10  OutDataTypeStr=Inherit: Inherit via back propagation
  Data Type Conversion1 : DataTypeConversion  OutDataTypeStr=int32  SaturateOnIntegerOverflow=off  RndMeth=Floor
  Data Type Conversion2 : DataTypeConversion  OutDataTypeStr=single  SaturateOnIntegerOverflow=off  RndMeth=Floor
  Data Type Conversion3 : DataTypeConversion  OutDataTypeStr=int32  SaturateOnIntegerOverflow=off  RndMeth=Floor
  Mux : Mux  Inputs=2
  PayLoad : etargetslib/Byte Pack  datatypes={'int32','int32','single'}  byteAlign=8
  checksum : Constant  Value=1234567897  OutDataTypeStr=Inherit: Inherit via back propagation
  PX4SILIntFloat : Outport  OutDataTypeStr=uint8  PortDimensions=120  VectorParamsAs1DForOutWhenUnconnected=off
  wires:
  inSILFloats/1 -> Data Type Conversion2/1
  inSILInts/1 -> Data Type Conversion1/1
  PayLoad/1 -> PX4SILIntFloat/1
  Data Type Conversion1/1 -> PayLoad/2
  Data Type Conversion2/1 -> PayLoad/3
  checksum/1 -> Mux/1
  Mux/1 -> Data Type Conversion3/1
  Data Type Conversion3/1 -> PayLoad/1
  CopterID/1 -> Mux/2

== system AirRefueling_Platform_ch10_WindGust/3D rendering engine/Subsystem1 ==
  copterID : Inport  PortDimensions=1
  vehicleType : Inport  Port=2  PortDimensions=1
  PosE : Inport  Port=3  PortDimensions=3
  AngEuler : Inport  Port=4  PortDimensions=3
  VelE : Inport  Port=5  PortDimensions=3
  Clock : Clock
  Constant1 : Constant  Value=[0,0,0,0]
  Constant3 : Constant  Value=[0,0,0]
  Constant4 : Constant  Value=[0,0,0]
  Constant5 : Constant  Value=[0,0,0]
  MotorPWMs1 : Constant  Value=[1000,1000,1000,1000,0,0,0,0]
  Subsystem : Subsystem
  toUnReal : Outport  VectorParamsAs1DForOutWhenUnconnected=off
  wires:
  VelE/1 -> Subsystem/4("VelE ")
  PosE/1 -> Subsystem/5(PosE)
  vehicleType/1 -> Subsystem/2(vehicleType)
  Clock/1 -> Subsystem/3(runnedTime)
  Constant4/1 -> Subsystem/10(RateB)
  Constant5/1 -> Subsystem/11(PosGPS)
  AngEuler/1 -> Subsystem/6(AngEuler)
  Subsystem/1(toUnReal) -> toUnReal/1
  Constant3/1 -> Subsystem/9(AccB)
  Constant1/1 -> Subsystem/7(AngQuatern)
  copterID/1 -> Subsystem/1(copterID)
  MotorPWMs1/1 -> Subsystem/8(MotorRPMS)

== system AirRefueling_Platform_ch10_WindGust/3D rendering engine/VehicleAttatchreq ==
  note: struct VehicleAttatch25 {
      | 	int checksum;//1234567892
      | 	int CopterIDs[25];
      | 	int AttatchIDs[25];
      | 	int AttatchTypes[25];//0：正常模式，1：相对位置不相对姿态，2：相对位置+偏航（不相对俯仰和滚转），3：相对位置+全姿态（俯仰滚转偏航）
      | }
  CopterIDs : Inport  PortDimensions=25
  AttatchIDs : Inport  Port=2  PortDimensions=25
  AttatchTypes : Inport  Port=3  PortDimensions=25
  Constant7 : Constant  Value=1234567892
  Data Type Conversion{,1..2,4} (4 alike) : DataTypeConversion  OutDataTypeStr=int32  SaturateOnIntegerOverflow=off  RndMeth=Floor
  PayLoad : etargetslib/Byte Pack  datatypes={'int32','int32','int32','int32'}  byteAlign=4
  Out1 : Outport  VectorParamsAs1DForOutWhenUnconnected=off
  wires:
  Data Type Conversion1/1 -> PayLoad/3
  AttatchTypes/1 -> Data Type Conversion2/1
  Data Type Conversion2/1 -> PayLoad/4
  PayLoad/1 -> Out1/1
  AttatchIDs/1 -> Data Type Conversion1/1
  Data Type Conversion/1 -> PayLoad/2
  CopterIDs/1 -> Data Type Conversion/1
  Constant7/1 -> Data Type Conversion4/1
  Data Type Conversion4/1 -> PayLoad/1

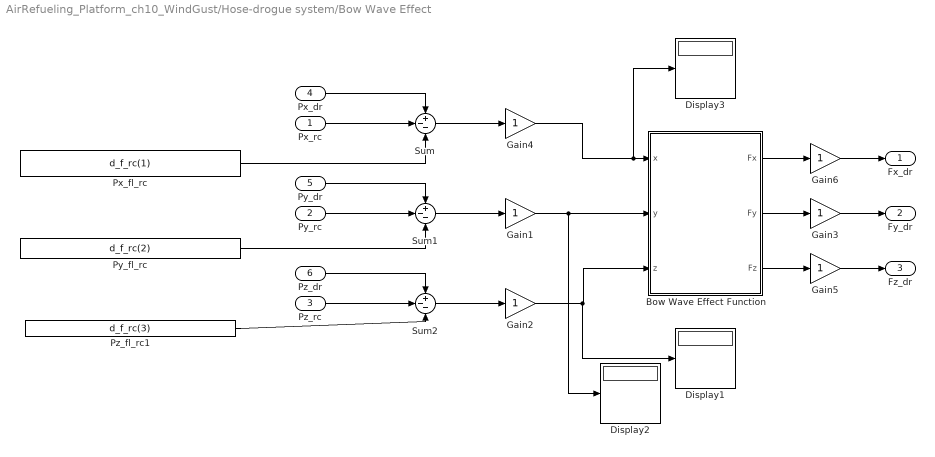
== system AirRefueling_Platform_ch10_WindGust/Hose-drogue system/Bow Wave Effect ==
  Px_rc : Inport
  Py_rc : Inport  Port=2
  Pz_rc : Inport  Port=3
  Px_dr : Inport  Port=4
  Py_dr : Inport  Port=5
  Pz_dr : Inport  Port=6
  Bow Wave Effect Function : MATLAB Function  TreatAsAtomicUnit=on
  Display1 : Display
  Display2 : Display
  Display3 : Display
  Gain{1..6} (6 alike) : Gain
  Px_fl_rc : Constant  Value=d_f_rc(1)
  Py_fl_rc : Constant  Value=d_f_rc(2)
  Pz_fl_rc1 : Constant  Value=d_f_rc(3)
  Sum : Sum  Inputs=+--
  Sum1 : Sum  Inputs=+--
  Sum2 : Sum  Inputs=+--
  Fx_dr : Outport
  Fy_dr : Outport  Port=2
  Fz_dr : Outport  Port=3
  wires:
  Sum2/1 -> Gain2/1
  Sum1/1 -> Gain1/1
  Bow Wave Effect Function/3(Fz) -> Gain5/1
  Bow Wave Effect Function/2(Fy) -> Gain3/1
  Bow Wave Effect Function/1(Fx) -> Gain6/1
  Gain6/1 -> Fx_dr/1
  Gain5/1 -> Fz_dr/1
  Gain3/1 -> Fy_dr/1
  Gain2/1 -> Display1/1, Bow Wave Effect Function/3(z)
  Gain1/1 -> Display2/1, Bow Wave Effect Function/2(y)
  Gain4/1 -> Display3/1, Bow Wave Effect Function/1(x)
  Pz_dr/1 -> Sum2/1
  Pz_fl_rc1/1 -> Sum2/3
  Pz_rc/1 -> Sum2/2
  Py_fl_rc/1 -> Sum1/3
  Py_dr/1 -> Sum1/1
  Py_rc/1 -> Sum1/2
  Px_dr/1 -> Sum/1
  Px_fl_rc/1 -> Sum/3
  Px_rc/1 -> Sum/2
  Sum/1 -> Gain4/1

== system AirRefueling_Platform_ch10_WindGust/Hose-drogue system/Collision Detection ==
  note: 这里的结果和发送坐标相同
  note: 相对距离
  note: 椎管的位置
  note: 椎管的速度
  note: 相对速度
  Pos_rc2tx : Inport
  Pos_dr : Inport  Port=2
  Constant : Constant  Value=d_pr_rc
  Constant1 : Constant  Value=Mdr
  Derivative : Derivative
  Derivative1 : Derivative
  Display1 : Display
  Display6 : Display
  MATLAB Function1 : MATLAB Function  TreatAsAtomicUnit=on
  Scope1 : Scope
  Scope2 : Scope
  Scope3 : Scope
  Sum1 : Sum  Inputs=|+-+
  Sum2 : Sum  Inputs=|++
  Sum3 : Sum  Inputs=|+-
  Sum5 : Sum  Inputs=|++
  drogue_delta_pos : Constant  Value=[0,0,0.04]
  修正数据让对接时误差为0 : Constant  Value=visual_err
  y : Outport
  wires:
  MATLAB Function1/1(F) -> Scope3/1, y/1
  Constant/1 -> Sum2/1
  Derivative/1 -> Sum3/1, MATLAB Function1/2(V_pr)
  Derivative1/1 -> Sum3/2, MATLAB Function1/4(V_dr)
  Constant1/1 -> MATLAB Function1/5(Mdr)
  Sum1/1 -> Display6/1, Scope1/1
  Sum3/1 -> Display1/1, Scope2/1
  Sum2/1 -> Derivative/1, Sum1/2, MATLAB Function1/1(Pos_pr)
  Sum5/1 -> Sum1/3, MATLAB Function1/3(Pos_dr), Derivative1/1
  Pos_dr/1 -> Sum5/1
  drogue_delta_pos/1 -> Sum5/2
  Pos_rc2tx/1 -> Sum2/2
  修正数据让对接时误差为0/1 -> MATLAB Function1/6(visual_err), Sum1/1

== system AirRefueling_Platform_ch10_WindGust/Hose-drogue system/DRdynamics ==
  Fx_dr : Inport
  Fy_dr : Inport  Port=2
  Fz_dr : Inport  Port=3
  Tanker_States : Inport  Port=4
  Demux : Demux  Outputs=3
  Demux1 : Demux  Outputs=3
  HDU : Subsystem
  Hose-Drogue1 : Subsystem
  Memory : Memory  InitialCondition=T_reel_initial
  Mux1 : Mux  Inputs=3
  Scope1 : Scope
  Scope2 : Scope
  Scope38 : Scope
  To Workspace1 : ToWorkspace  VariableName=dl_1  SampleTime=-1
  To Workspace2 : ToWorkspace  VariableName=ddl_1  SampleTime=-1
  To Workspace3 : ToWorkspace  VariableName=T_hose  SampleTime=-1
  length2 : Constant  Value=zeros(3,N)
  Pxdr_tk : Outport
  Pydr_tk : Outport  Port=2
  Pzdr_tk : Outport  Port=3
  plink : Outport  Port=4
  wires:
  Demux1/1 -> Hose-Drogue1/1(pt)
  Demux1/2 -> Hose-Drogue1/2(vt)
  Demux1/3 -> Hose-Drogue1/3(at)
  length2/1 -> Hose-Drogue1/4(w)
  Hose-Drogue1/2(t) -> Scope38/1, Memory/1, To Workspace3/1
  Memory/1 -> HDU/1(t_hose)
  HDU/1(l_1) -> Hose-Drogue1/5(link length)
  HDU/3(ddl_1) -> Hose-Drogue1/7(DD link length), Scope2/1, To Workspace2/1
  Hose-Drogue1/1(p link) -> plink/1
  Mux1/1 -> Hose-Drogue1/8(Fb)
  Fx_dr/1 -> Mux1/1
  Fy_dr/1 -> Mux1/2
  Fz_dr/1 -> Mux1/3
  Hose-Drogue1/3(pdr) -> Demux/1
  Demux/1 -> Pxdr_tk/1
  Demux/2 -> Pydr_tk/1
  Demux/3 -> Pzdr_tk/1
  Tanker_States/1 -> Demux1/1
  HDU/2(dl_1) -> To Workspace1/1, Scope1/1, Hose-Drogue1/6(D link length)

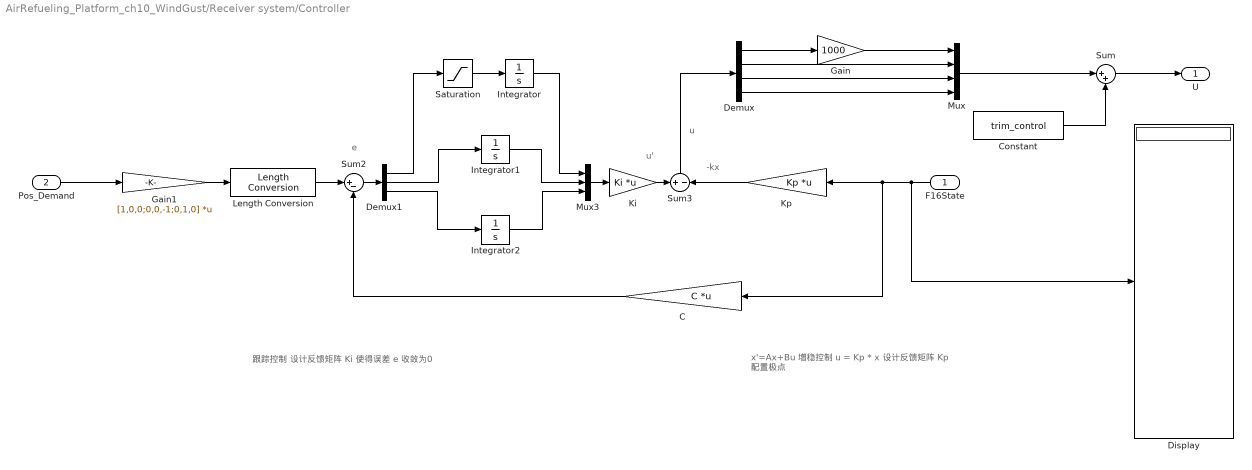
== system AirRefueling_Platform_ch10_WindGust/Receiver system/Controller ==
  note: u
  note: -kx
  note: u'
  note: e
  note: 跟踪控制
      | 设计反馈矩阵 Ki 使得误差 e 收敛为0
  note: x'=Ax+Bu
      | 增稳控制 u = Kp * x
      | 设计反馈矩阵 Kp 配置极点
  F16State : Inport
  Pos_Demand : Inport  Port=2
  C : Gain  Gain=C  Multiplication=Matrix(K*u) (u vector)
  Constant : Constant  Value=trim_control
  Demux : Demux
  Demux1 : Demux  Outputs=3
  Display : Display
  Gain : Gain  Gain=1000
  Gain1 : Gain  Gain=[1,0,0;0,0,-1;0,1,0]  Multiplication=Matrix(K*u) (u vector)
  Integrator : Integrator
  Integrator1 : Integrator
  Integrator2 : Integrator
  Ki : Gain  Gain=Ki  Multiplication=Matrix(K*u) (u vector)
  Kp : Gain  Gain=Kp  Multiplication=Matrix(K*u) (u vector)
  Length Conversion : aerolibconvert2/Length Conversion  IU=m  OU=ft
  Mux : Mux
  Mux3 : Mux  Inputs=3
  Saturation : Saturate  UpperLimit=15  LowerLimit=-15
  Sum : Sum  Inputs=|++
  Sum2 : Sum  Inputs=|+-
  Sum3 : Sum  Inputs=+|-
  U : Outport
  wires:
  Sum2/1 -> Demux1/1
  C/1 -> Sum2/2
  Mux3/1 -> Ki/1
  Demux1/2 -> Integrator1/1
  F16State/1 -> Display/1, Kp/1, C/1
  Integrator1/1 -> Mux3/2
  Integrator/1 -> Mux3/1
  Demux1/3 -> Integrator2/1
  Integrator2/1 -> Mux3/3
  Length Conversion/1 -> Sum2/1
  Demux1/1 -> Saturation/1
  Ki/1 -> Sum3/1
  Kp/1 -> Sum3/2
  Sum3/1 -> Demux/1
  Saturation/1 -> Integrator/1
  Demux/2 -> Mux/2
  Demux/3 -> Mux/3
  Demux/4 -> Mux/4
  Demux/1 -> Gain/1
  Gain/1 -> Mux/1
  Pos_Demand/1 -> Gain1/1
  Gain1/1 -> Length Conversion/1
  Constant/1 -> Sum/2
  Mux/1 -> Sum/1
  Sum/1 -> U/1

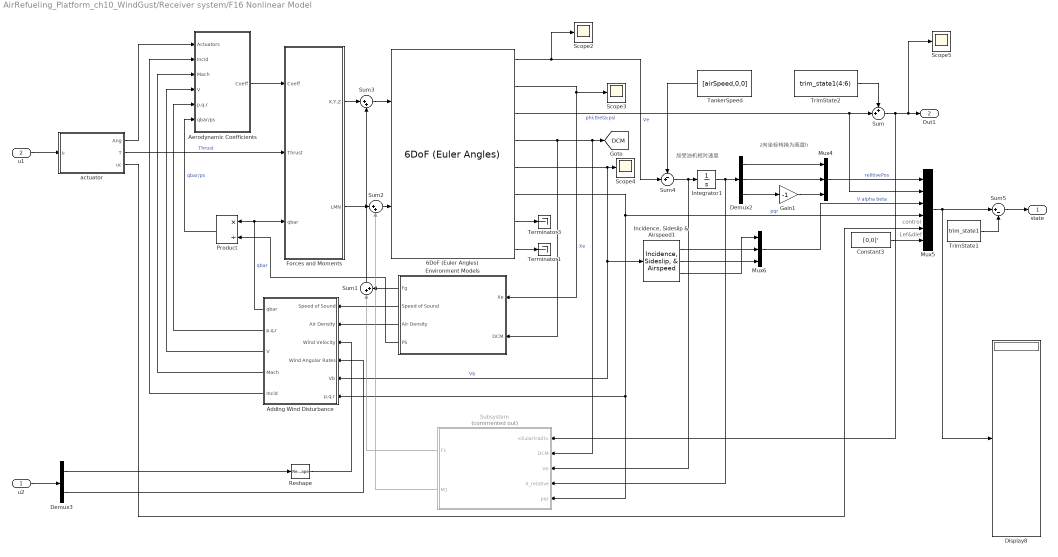
== system AirRefueling_Platform_ch10_WindGust/Receiver system/F16 Nonlinear Model ==
  note: 加受油机相对速度
  note: z向坐标转换为高度h
  note: Lef&dlef
  note: control
  u2 : Inport
  u1 : Inport  Port=2
  6DoF (Euler Angles) : aerolibobsolete/6DoF (Euler Angles)  units=English (Velocity in ft/s)  mtype=Fixed  rep=Euler Angles  xme_0=xyz_0  Vm_0=uvw_0  eul_0=Euler_0  pm_0=pqr_0  mass_0=mass  mass_e=0.5  mass_f=2.0  inertia=Inertia  inertia_e=eye(3)  inertia_f=2*eye(3)  k_quat=1.0
      settings: SourceProductBaseCode=AE
  Adding Wind Disturbance : Subsystem
  Aerodynamic Coefficients : Subsystem
  Constant3 : Constant  Value=[0,0]'
  Demux2 : Demux  Outputs=3
  Demux3 : Demux  Outputs=2
  Display8 : Display
  Environment Models : Subsystem
  Forces and Moments : Subsystem
  Gain1 : Gain  Gain=-1
  "Incidence, Sideslip & Airspeed1" : aerolibasang/Incidence, Sideslip, & Airspeed
  Integrator1 : Integrator
  Mux4 : Mux  Inputs=3
  Mux5 : Mux  Inputs=6
  Mux6 : Mux  Inputs=3
  Product : Product  Inputs=*/  InputSameDT=on  SaturateOnIntegerOverflow=on  OutDataTypeStr=Inherit: Same as first input
  Reshape : Reshape
  Scope{2..5} (4 alike) : Scope
  Subsystem : Subsystem  Commented=on
  Sum : Sum  Inputs=++|
  Sum1 : Sum  Inputs=|++  InputSameDT=on  SaturateOnIntegerOverflow=on  OutDataTypeStr=Inherit: Same as first input
  Sum2 : Sum  Inputs=|++  InputSameDT=on  SaturateOnIntegerOverflow=on  OutDataTypeStr=Inherit: Same as first input
  Sum3 : Sum  Inputs=|++  InputSameDT=on  SaturateOnIntegerOverflow=on  OutDataTypeStr=Inherit: Same as first input
  Sum4 : Sum  Inputs=-+|
  Sum5 : Sum  Inputs=|+-
  TankerSpeed : Constant  Value=[airSpeed,0,0]
  Terminator1 : Terminator
  Terminator3 : Terminator
  TrimState1 : Constant  Value=trim_state1
  TrimState2 : Constant  Value=trim_state1(4:6)
  actuator : Subsystem
  state : Outport
  Out1 : Outport  Port=2
  tag scope: DCM=global
  wires:
  6DoF (Euler Angles)/8 -> Terminator1/1
  6DoF (Euler Angles)/7 -> Terminator3/1
  Adding Wind Disturbance/5(Incid) -> Aerodynamic Coefficients/2(Incid)
  Aerodynamic Coefficients/1(Coeff) -> Forces and Moments/1(Coeff)
  Environment Models/2(Speed of Sound) -> Adding Wind Disturbance/1(Speed of Sound)
  Environment Models/3(Air Density) -> Adding Wind Disturbance/2(Air Density)
  Adding Wind Disturbance/1(qbar) -> Forces and Moments/3(qbar), Product/1  "qbar"
  Forces and Moments/1(X,Y,Z) -> Sum3/1
  Sum3/1 -> 6DoF (Euler Angles)/1
  Adding Wind Disturbance/3(V) -> Aerodynamic Coefficients/4(V)
  Adding Wind Disturbance/4(Mach) -> Aerodynamic Coefficients/3(Mach)
  Adding Wind Disturbance/2("p,q,r ") -> Aerodynamic Coefficients/5(p,q,r)
  Environment Models/4(PS) -> Product/2
  Product/1 -> Aerodynamic Coefficients/6(qbar/ps)  "qbar/ps"
  u1/1 -> actuator/1(u)
  actuator/2(T) -> Forces and Moments/2(Thrust)  "Thrust"
  actuator/1(Ang) -> Aerodynamic Coefficients/1(Actuators)
  6DoF (Euler Angles)/3 -> Mux5/2, Sum/2  "phi;theta;psi"
  "Incidence, Sideslip & Airspeed1"/1 -> Mux6/2
  "Incidence, Sideslip & Airspeed1"/2 -> Mux6/3
  Mux6/1 -> Mux5/3  "V alpha beta"
  "Incidence, Sideslip & Airspeed1"/3 -> Mux6/1
  6DoF (Euler Angles)/6 -> Subsystem/5(pqr), Adding Wind Disturbance/6(p,q,r), Mux5/4  "pqr"
  6DoF (Euler Angles)/5 -> Scope4/1, Adding Wind Disturbance/5(Vb), "Incidence, Sideslip & Airspeed1"/1  "Vb"
  Mux5/1 -> Display8/1, Sum5/1
  TrimState1/1 -> Sum5/2
  Sum5/1 -> state/1
  actuator/3(uc) -> Mux5/5
  Constant3/1 -> Mux5/6
  Demux2/2 -> Mux4/2
  Demux2/3 -> Gain1/1
  Mux4/1 -> Mux5/1  "relitivePos"
  Demux2/1 -> Mux4/1
  Gain1/1 -> Mux4/3
  Sum4/1 -> Subsystem/3(Ve), Integrator1/1
  Integrator1/1 -> Subsystem/4(X_relative), Demux2/1
  6DoF (Euler Angles)/2 -> Scope3/1, Environment Models/1(Xe)  "Xe"
  u2/1 -> Demux3/1
  Reshape/1 -> Adding Wind Disturbance/3(Wind Velocity)
  Demux3/1 -> Reshape/1
  Demux3/2 -> Adding Wind Disturbance/4(Wind Angular Rates)
  TrimState2/1 -> Sum/1
  6DoF (Euler Angles)/1 -> Scope2/1, Sum4/2  "Ve"
  TankerSpeed/1 -> Sum4/1
  Sum/1 -> Subsystem/1(<Eular(rad)>), Scope5/1, Out1/1
  6DoF (Euler Angles)/4 -> Environment Models/2(DCM), [DCM], Subsystem/2(DCM)
  Environment Models/1(Fg) -> Sum1/2
  Subsystem/1(F1) -> Sum1/1
  Sum1/1 -> Sum3/2
  Forces and Moments/2(LMN) -> Sum2/1
  Sum2/1 -> 6DoF (Euler Angles)/2
  Subsystem/2(M1) -> Sum2/2
